simulink model "Rasterung_Current_Voltage"  (R2015a)
settings: Solver=FixedStepDiscrete  SolverMode=SingleTasking  StartTime=0.0  StopTime=100  FixedStep=1e-3  RelTol=1e-3
libraries: mbed_spi_power x8, mbed_lib x4
settings Model: Creator=svenl  LastModifiedBy=oh
settings OptimizationCC: OptimizeModelRefInitCode=on  LifeSpan=1
settings HardwareCC: ProdLargestAtomicInteger=Long  ProdLargestAtomicFloat=Double  ProdEndianess=LittleEndian  ProdHWDeviceType=ARM Compatible->ARM Cortex
settings RTWCC: SystemTargetFile=mbed.tlc  TemplateMakefile=mbed.tmf  Description=Mbed Target (Embedded Target)  TargetLang=C++
settings CodeAppCC: IgnoreCustomStorageClasses=off
settings STFCustomTargetCC: CombineOutputUpdateFcns=on  SupportContinuousTime=off  SupportVariableSizeSignals=off  SystemTargetFile=mbed.tlc
settings ERTTargetCC: SupportContinuousTime=off  SupportVariableSizeSignals=off  ERTCustomFileTemplate=mbed_file_process.tlc

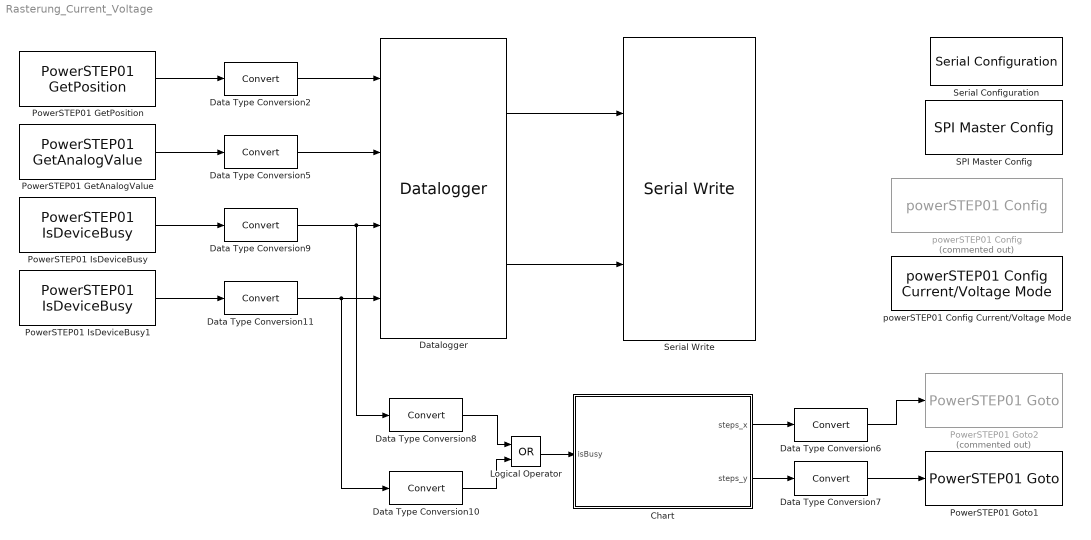
== system Rasterung_Current_Voltage ==
  Chart : Stateflow chart  TreatAsAtomicUnit=on
  Data Type Conversion{2,5..11} (8 alike) : DataTypeConversion
  Datalogger : mbed_lib/Utilities/Datalogger  TypeInputPorts={ 'int32' 1 'int32' 1 'int32' 1 'int32' 1 }  TypeOfInputs={'1*int32' '1*int32' '1*int32' '1*int32'}  BufferSize=100  errEn=off  SampleTime=-1
  Logical Operator : Logic  Operator=OR  AllPortsSameDT=off  OutDataTypeStr=boolean
  PowerSTEP01 GetAnalogValue : mbed_spi_power/PowerSTEP01 GetAnalogValue  SPINr=1  NumMotors=1  SSELPort=B  SSELPin=6  SampleTime=0.1  Parameter_C=POWERSTEP01_ABS_POS  Parameter_V=POWERSTEP01_ABS_POS
  PowerSTEP01 GetPosition : mbed_spi_power/PowerSTEP01 GetPosition  SPINr=1  NumMotors=2  SSELPort=B  SSELPin=6  SampleTime=0.1
  PowerSTEP01 Goto1 : mbed_spi_power/PowerSTEP01 Goto  SPINr=1  NumMotors=2  SSELPort=B  SSELPin=6  SampleTime=-1
  PowerSTEP01 Goto2 : mbed_spi_power/PowerSTEP01 Goto  Commented=on  SPINr=1  NumMotors=1  SSELPort=B  SSELPin=6  SampleTime=-1
  PowerSTEP01 IsDeviceBusy : mbed_spi_power/PowerSTEP01 IsDeviceBusy  SPINr=1  NumMotors=1  SSELPort=B  SSELPin=6  SampleTime=-1
  PowerSTEP01 IsDeviceBusy1 : mbed_spi_power/PowerSTEP01 IsDeviceBusy  SPINr=1  NumMotors=2  SSELPort=B  SSELPin=6  SampleTime=-1
  SPI Master Config : mbed_lib/SPI/SPI Master Config  Priority=0  SpiPort=1  SpiFreq=100000  MosiPort=A  MosiPin=7  MisoPort=A  MisoPin=6  SclkPort=A  SclkPin=5
  Serial Configuration : mbed_lib/Serial/Serial Configuration  SerialPort=1  TXPort=A  TXPin=2  RXPort=A  RXPin=3  BaudRate=9600
  Serial Write : mbed_lib/Serial/Serial Write  SerialPort=1  numData=on  SampleTime=-1
  powerSTEP01 Config : mbed_spi_power/powerSTEP01 Config  Priority=0  Commented=on  SPINr=1  SSELPort=B  SSELPin=6  ResetPort=A  ResetPin=9  ACC=50  DEC=50  MaxSpeed=200  MinSpeed=0  FullStepSpeed=150  Overcurrent=100  StepMode=STEP_MODE_1_128  Holdtorque=20  Runtorque=20  ACCtorque=20  DECtorque=20  Motor2SEL=on  ACC_1=50  DEC_1=50  MaxSpeed_1=500  MinSpeed_1=0  FullStepSpeed_1=350  Overcurrent_1=150  StepMode_1=STEP_MODE_1_32  Holdtorque_1=50  Runtorque_1=50  ACCtorque_1=50  DECtorque_1=50  Motor3SEL=off  ACC_2=0  DEC_2=0  MaxSpeed_2=0  MinSpeed_2=0  FullStepSpeed_2=0  Overcurrent_2=0  StepMode_2=STEP_MODE_FULL  Holdtorque_2=0  Runtorque_2=0  ACCtorque_2=0  DECtorque_2=0
  powerSTEP01 Config Current/Voltage Mode : mbed_spi_power/powerSTEP01 Config Current//Voltage Mode  Priority=0  SPINr=1  SSELPort=B  SSELPin=6  ResetPort=A  ResetPin=15  ACC=12  DEC=12  MaxSpeed=300  MinSpeed=0  FullStepSpeed=250  Overcurrent=100  StepMode=STEP_MODE_1_128  VC_Mode1=on  Holdtorque=50  Runtorque=50  ACCtorque=50  DECtorque=50  Motor2SEL=on  ACC_1=12  DEC_1=12  MaxSpeed_1=300  MinSpeed_1=0  FullStepSpeed_1=250  Overcurrent_1=100  StepMode_1=STEP_MODE_FULL  VC_Mode2=off  Holdtorque_1=50  Runtorque_1=50  ACCtorque_1=50  DECtorque_1=50  Motor3SEL=off  ACC_2=0  DEC_2=0  MaxSpeed_2=0  MinSpeed_2=0  FullStepSpeed_2=0  Overcurrent_2=0  StepMode_2=STEP_MODE_FULL  VC_Mode3=off  Holdtorque_2=0  Runtorque_2=0  ACCtorque_2=0  DECtorque_2=0
  wires:
  Datalogger/1 -> Serial Write/1
  Datalogger/2 -> Serial Write/2
  PowerSTEP01 GetPosition/1 -> Data Type Conversion2/1
  Data Type Conversion2/1 -> Datalogger/1
  PowerSTEP01 GetAnalogValue/1 -> Data Type Conversion5/1
  Data Type Conversion5/1 -> Datalogger/2
  Chart/2(steps_y) -> Data Type Conversion7/1
  Chart/1(steps_x) -> Data Type Conversion6/1
  Data Type Conversion6/1 -> PowerSTEP01 Goto2/1
  Data Type Conversion7/1 -> PowerSTEP01 Goto1/1
  Data Type Conversion8/1 -> Logical Operator/1
  Data Type Conversion10/1 -> Logical Operator/2
  Data Type Conversion9/1 -> Data Type Conversion8/1, Datalogger/3
  PowerSTEP01 IsDeviceBusy/1 -> Data Type Conversion9/1
  PowerSTEP01 IsDeviceBusy1/1 -> Data Type Conversion11/1
  Data Type Conversion11/1 -> Data Type Conversion10/1, Datalogger/4
  Logical Operator/1 -> Chart/1(isBusy)

== stateflow chart Rasterung_Current_Voltage/Chart ==
  state Init
    entry:
    steps_x=0;
    steps_y=0;
  state y_Bewegung
    entry:
    steps_y=0;
  state y_Bewegung1
    entry:
    steps_y=1000;
  state x_Bewegung1
    entry: steps_x= 0;
  state x_Bewegung
    entry: steps_x=steps_x + 500;
  (default) -> Init
  Init -> y_Bewegung
  (junction 12) -> y_Bewegung1 [order 1] : [steps_y==0]
  y_Bewegung1 -> (junction 18) : after(1,sec)[isBusy==0]
  y_Bewegung -> (junction 18) : after(1,sec)[isBusy==0]
  (junction 12) -> y_Bewegung [order 2] : [steps_y==1000]
  x_Bewegung1 -> (junction 12) : after(1,sec)[isBusy==0]
  x_Bewegung -> (junction 12) : after(1,sec)[isBusy==0]
  (junction 18) -> x_Bewegung [order 2] : [steps_x<5001]
  (junction 18) -> x_Bewegung1 [order 1] : [steps_x>5000]
  data: steps_x output double; steps_y output double; isBusy input
